simulink model "hev_parallel"  (R2015b)
settings: Solver=VariableStepAuto  StartTime=0.0  StopTime=100  RelTol=1e-3
undefined symbols (not defined in the file): A, C, f, g, M, p, Vw
libraries: simulink x3
settings Model: Creator=ihong-gyu  LastModifiedBy=ihong-gyu
settings SolverCC: ZeroCrossControl=EnableAll

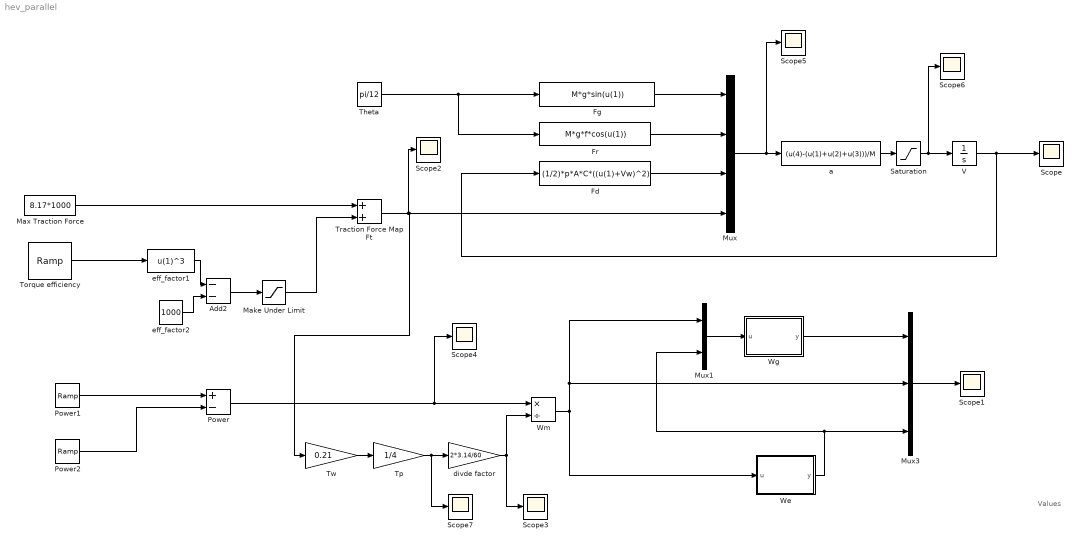
== system hev_parallel ==
  note: Values
  Add2 : Sum  Inputs=--
  Fd : Fcn  Expr=(1/2)*p*A*C*((u(1)+Vw)^2)
  Fg : Fcn  Expr=M*g*sin(u(1))
  Fr : Fcn  Expr=M*g*f*cos(u(1))
  Make Under Limit : Saturate  UpperLimit=0  LowerLimit=-1000
  Max Traction Force : Constant  Value=8.17*1000
  Mux : Mux
  Mux1 : Mux  Inputs=2
  Mux3 : Mux  Inputs=3
  Power : Sum  Inputs=+-
  Power1 : simulink/Sources/Ramp  slope=3000  start=0  X0=0
  Power2 : simulink/Sources/Ramp  slope=3000  start=20  X0=0
  Saturation : Saturate  UpperLimit=100000000  LowerLimit=0
  Scope{,1..7} (8 alike) : Scope
  Theta : Constant  Value=pi/12
  Torque efficiency : simulink/Sources/Ramp  slope=0.5  start=20  X0=-1000^(1/3)
  Tp : Gain  Gain=1/4
  Traction Force Map Ft : Sum
  Tw : Gain  Gain=0.21
  V : Integrator
  We : MATLAB Function  TreatAsAtomicUnit=on
  Wg : MATLAB Function  TreatAsAtomicUnit=on
  Wm : Product  Inputs=*/
  a : Fcn  Expr=(u(4)-(u(1)+u(2)+u(3)))/M
  divde factor : Gain  Gain=2*3.14/60
  eff_factor1 : Fcn  Expr=u(1)^3
  eff_factor2 : Constant  Value=1000
  wires:
  Fg/1 -> Mux/1
  Fr/1 -> Mux/2
  Fd/1 -> Mux/3
  Mux/1 -> Scope5/1, a/1
  V/1 -> Fd/1, Scope/1
  Theta/1 -> Fr/1, Fg/1
  Max Traction Force/1 -> Traction Force Map Ft/1
  eff_factor1/1 -> Add2/1
  eff_factor2/1 -> Add2/2
  Traction Force Map Ft/1 -> Tw/1, Mux/4, Scope2/1
  Power1/1 -> Power/1
  Power2/1 -> Power/2
  Power/1 -> Scope4/1, Wm/1
  Wm/1 -> We/1(u), Mux1/1, Mux3/2
  Mux1/1 -> Wg/1(u)
  We/1(y) -> Mux3/3, Mux1/2
  Wg/1(y) -> Mux3/1
  Mux3/1 -> Scope1/1
  Tw/1 -> Tp/1
  Tp/1 -> divde factor/1, Scope7/1
  divde factor/1 -> Wm/2, Scope3/1
  Torque efficiency/1 -> eff_factor1/1
  Saturation/1 -> Scope6/1, V/1
  a/1 -> Saturation/1
  Add2/1 -> Make Under Limit/1
  Make Under Limit/1 -> Traction Force Map Ft/2

== matlab function hev_parallel/Wg ==
  data: u input; y output
function y = fcn(u)
%#codegen

R = 20/60;

y = ((1+R)*u(2)-u(1))/R;

== matlab function hev_parallel/We ==
  data: u input; y output
function y = fcn(u)
%#codegen

if(u<1000)
    y=0;
else
    y=2000;
end
